simulink model "nicht_linear_model"  (R2019a)
settings: Solver=VariableStepAuto  StartTime=0.0  StopTime=10.0  RelTol=1e-3
values from neighbouring files (symbols this model uses):
  b = 0.1    [inv_pend.m]
  g = 9.8    [inv_pend.m]
  I = 0.006    [inv_pend.m]
  l = 0.3    [inv_pend.m]
  m = 0.5    [inv_pend.m]
  M = 0.5    [inv_pend.m]
settings Model: Creator=Naveen  LastModifiedBy=Naveen

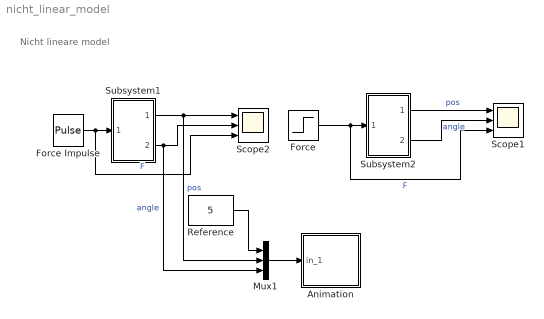
== system nicht_linear_model ==
  note: Nicht lineare model
  Animation : Subsystem  mask(Pendulum plot){RefBlock=Reference}
      mask prompts: RefBlock "DC reference signal block name:"
      mask help: Pendulum plot
      mask Help: Pendulum animation function using Handle graphics.
      mask Display: plot([-10 10],[0 0],[-2 -2 2 2],[0 1 1 0],[0 3],[1 5])
  Force : Step  After=5  SampleTime=0
  Force Impulse : DiscretePulseGenerator  PulseType=Time based  Amplitude=100  Period=100  PulseWidth=0.01  PhaseDelay=3
  Mux1 : Mux  Inputs=3
  Reference : Constant  Value=5
  Scope1 : Scope  NumInputPorts=3
  Scope2 : Scope  NumInputPorts=3
  Subsystem1 : Subsystem
  Subsystem2 : Subsystem
  wires:
  Force Impulse/1 -> Scope2/3, Subsystem1/1(Force)  "F"
  Subsystem1/2(Angle) -> Mux1/3, Scope2/2  "angle"
  Force/1 -> Scope1/3, Subsystem2/1(Force)  "F"
  Subsystem2/1(Position) -> Scope1/1  "pos"
  Subsystem2/2(Angle) -> Scope1/2  "angle"
  Subsystem1/1(Position) -> Scope2/1, Mux1/2  "pos"
  Reference/1 -> Mux1/1
  Mux1/1 -> Animation/1(in_1)

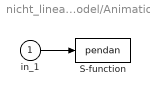
== system nicht_linear_model/Animation ==
  in_1 : Inport
  S-function : S-Function  FunctionName=pendan  Parameters=RefBlock  SFunctionDeploymentMode=off  EnableBusSupport=off
      settings: DeleteFcn=pendan([],[],[],'DeleteBlock');
  wires:
  in_1/1 -> S-function/1

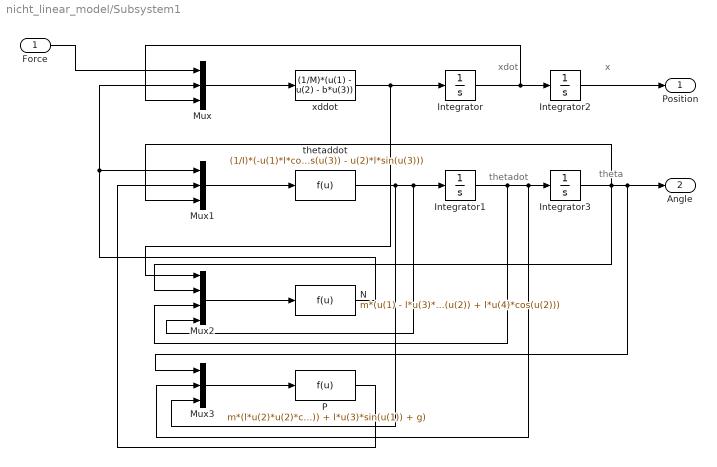
== system nicht_linear_model/Subsystem1 ==
  note: x
  note: thetadot
  note: theta
  note: xdot
  Force : Inport
  Integrator : Integrator  ContinuousStateAttributes='xdot'
  Integrator1 : Integrator  ContinuousStateAttributes='thetadot'
  Integrator2 : Integrator  ContinuousStateAttributes='x'
  Integrator3 : Integrator  ContinuousStateAttributes='theta'
  Mux : Mux  Inputs=3
  Mux1 : Mux  Inputs=3
  Mux2 : Mux
  Mux3 : Mux  Inputs=3
  N : Fcn  Expr=m*(u(1) - l*u(3)*u(3)*sin(u(2)) + l*u(4)*cos(u(2)))
  P : Fcn  Expr=m*(l*u(2)*u(2)*cos(u(1)) + l*u(3)*sin(u(1)) + g)
  thetaddot : Fcn  Expr=(1/I)*(-u(1)*l*cos(u(3)) - u(2)*l*sin(u(3)))
  xddot : Fcn  Expr=(1/M)*(u(1) - u(2) - b*u(3))
  Position : Outport
  Angle : Outport  Port=2
  wires:
  Integrator2/1 -> Position/1
  Integrator3/1 -> Mux2/2, Mux1/3, Angle/1, Mux3/1
  Mux3/1 -> P/1
  Force/1 -> Mux/1
  Integrator1/1 -> Mux2/3, Mux3/2, Integrator3/1
  xddot/1 -> Mux2/1, Integrator/1
  Integrator/1 -> Mux/3, Integrator2/1
  Mux1/1 -> thetaddot/1
  Mux2/1 -> N/1
  Mux/1 -> xddot/1
  N/1 -> Mux1/1, Mux/2
  thetaddot/1 -> Mux3/3, Mux2/4, Integrator1/1
  P/1 -> Mux1/2

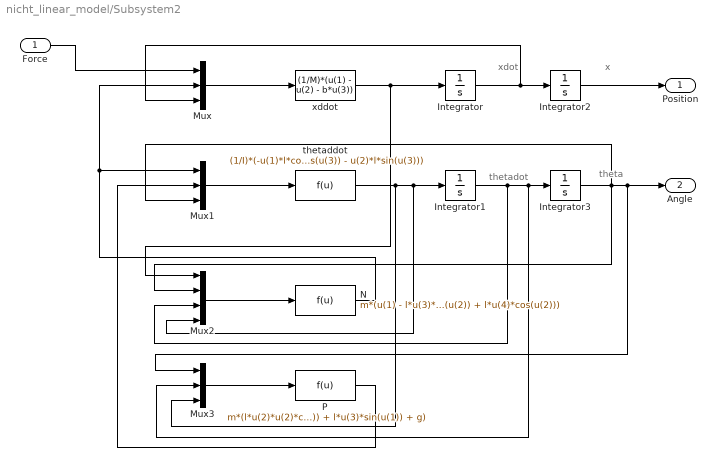
== system nicht_linear_model/Subsystem2 ==
  note: x
  note: thetadot
  note: theta
  note: xdot
  Force : Inport
  Integrator : Integrator  ContinuousStateAttributes='xdot'
  Integrator1 : Integrator  ContinuousStateAttributes='thetadot'
  Integrator2 : Integrator  ContinuousStateAttributes='x'
  Integrator3 : Integrator  ContinuousStateAttributes='theta'
  Mux : Mux  Inputs=3
  Mux1 : Mux  Inputs=3
  Mux2 : Mux
  Mux3 : Mux  Inputs=3
  N : Fcn  Expr=m*(u(1) - l*u(3)*u(3)*sin(u(2)) + l*u(4)*cos(u(2)))
  P : Fcn  Expr=m*(l*u(2)*u(2)*cos(u(1)) + l*u(3)*sin(u(1)) + g)
  thetaddot : Fcn  Expr=(1/I)*(-u(1)*l*cos(u(3)) - u(2)*l*sin(u(3)))
  xddot : Fcn  Expr=(1/M)*(u(1) - u(2) - b*u(3))
  Position : Outport
  Angle : Outport  Port=2
  wires:
  Integrator2/1 -> Position/1
  Integrator3/1 -> Mux2/2, Mux1/3, Angle/1, Mux3/1
  Mux3/1 -> P/1
  Force/1 -> Mux/1
  Integrator1/1 -> Mux2/3, Mux3/2, Integrator3/1
  xddot/1 -> Mux2/1, Integrator/1
  Integrator/1 -> Mux/3, Integrator2/1
  Mux1/1 -> thetaddot/1
  Mux2/1 -> N/1
  Mux/1 -> xddot/1
  N/1 -> Mux1/1, Mux/2
  thetaddot/1 -> Mux3/3, Mux2/4, Integrator1/1
  P/1 -> Mux1/2
